simulink model "model"  (R2020b)
settings: Solver=VariableStepAuto  StartTime=0.0  StopTime=10.0  RelTol=1e-3
undefined symbols (not defined in the file): Br, Bs, im, Js, km, Kr, Ks, m, rp
settings Model: DataDictionary=EPS_data_dic.sldd  Creator=Arvind Hishikar  LastModifiedBy=Arvind Hishikar

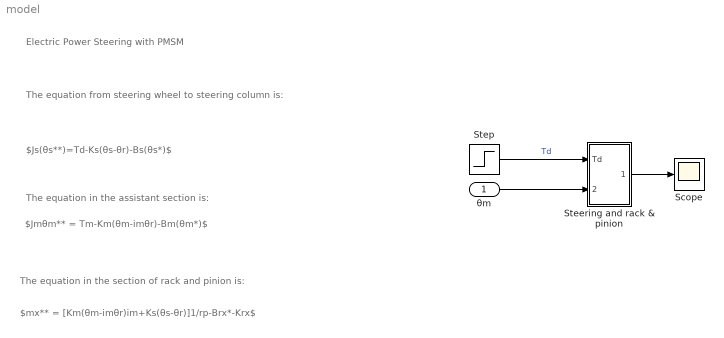
== system model ==
  note: Electric Power Steering with PMSM
  note: The equation in the section of rack and pinion is:
  note: The equation in the assistant section is:
  note: $mx** = [Km(θm-imθr)im+Ks(θs-θr)]1/rp-Brx*-Krx$
  note: $Jmθm** = Tm-Km(θm-imθr)-Bm(θm*)$
  note: The equation from steering wheel to steering column is:
  note: $Js(θs**)=Td-Ks(θs-θr)-Bs(θs*)$
  θm : Inport
  Scope : Scope
  Steering and rack & pinion : Subsystem
  Step : Step  SampleTime=0
  wires:
  Step/1 -> Steering and rack & pinion/1(Td)  "Td"
  θm/1 -> Steering and rack & pinion/2(θm)
  Steering and rack & pinion/1(Outport) -> Scope/1

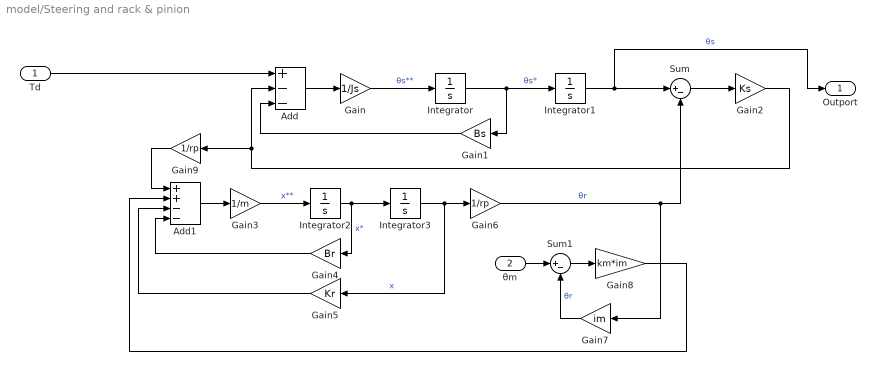
== system model/Steering and rack & pinion ==
  Td : Inport
  θm : Inport  Port=2
  Add : Sum  Inputs=+--
  Add1 : Sum  Inputs=++--
  Gain : Gain  Gain=1/Js
  Gain1 : Gain  Gain=Bs
  Gain2 : Gain  Gain=Ks
  Gain3 : Gain  Gain=1/m
  Gain4 : Gain  Gain=Br
  Gain5 : Gain  Gain=Kr
  Gain6 : Gain  Gain=1/rp
  Gain7 : Gain  Gain=im
  Gain8 : Gain  Gain=km*im
  Gain9 : Gain  Gain=1/rp
  Integrator{,1..3} (4 alike) : Integrator
  Sum : Sum  Inputs=|+-
  Sum1 : Sum  Inputs=|+-
  Outport : Outport
  wires:
  Gain5/1 -> Add1/3
  Gain/1 -> Integrator/1  "θs**"
  Gain6/1 -> Sum/2, Gain7/1  "θr"
  Integrator3/1 -> Gain6/1, Gain5/1  "x"
  Add1/1 -> Gain3/1
  Integrator2/1 -> Gain4/1, Integrator3/1  "x*"
  θm/1 -> Sum1/1
  Gain8/1 -> Add1/2
  Gain4/1 -> Add1/4
  Gain2/1 -> Gain9/1, Add/2
  Integrator/1 -> Gain1/1, Integrator1/1  "θs*"
  Gain3/1 -> Integrator2/1  "x**"
  Sum1/1 -> Gain8/1
  Sum/1 -> Gain2/1
  Gain1/1 -> Add/3
  Td/1 -> Add/1
  Gain7/1 -> Sum1/2  "θr"
  Add/1 -> Gain/1
  Gain9/1 -> Add1/1
  Integrator1/1 -> Outport/1, Sum/1  "θs"
